simulink model "proj7_p1"  (R2016b)
settings: Solver=VariableStepAuto  StartTime=0.0  StopTime=10.0  RelTol=1e-3  EnableMultiTasking=on
undefined symbols (not defined in the file or in its folder): mc
settings Model: Creator=dave0651  LastModifiedBy=Jinesh
settings OptimizationCC: LifeSpan=inf
settings DebuggingCC: SFUnexpectedBacktrackingDiag=warning  SFNoUnconditionalDefaultTransitionDiag=warning  SFExecutionAtInitializationDiag=none
settings GRTTargetCC: TargetLangStandard=C89/C90 (ANSI)  GeneratePreprocessorConditionals=Disable all
settings ConfigComp: CovMetricSettings=dw  CovHtmlReporting=on  CovSaveCumulativeToWorkspaceVar=on  CovSaveSingleToWorkspaceVar=on  CovExternalEMLEnable=off

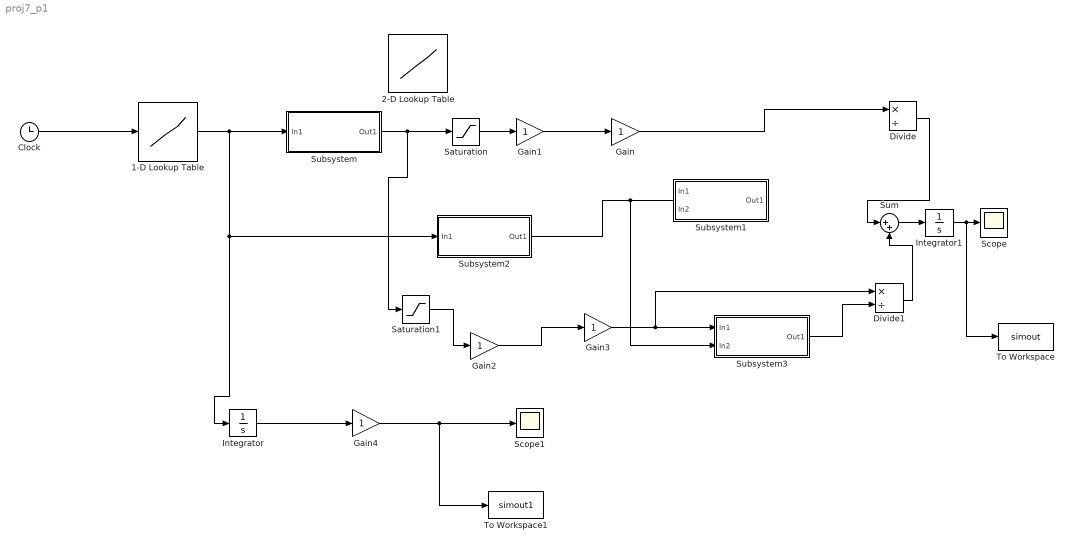
== system proj7_p1 ==
  1-D Lookup Table : Lookup_n-D  NumberOfTableDimensions=1  BreakpointsForDimension1=[-5:5]  Table=tanh([-5:5])  InternalRulePriority=Speed  RndMeth=Simplest  InputSameDT=on
  2-D Lookup Table : Lookup_n-D  BreakpointsForDimension1=[1:3]  BreakpointsForDimension2=[1:3]  InternalRulePriority=Speed  RndMeth=Simplest  InputSameDT=on
  Clock : Clock
  Divide : Product  Inputs=*/
  Divide1 : Product  Inputs=*/
  Gain{,1..4} (5 alike) : Gain
  Integrator : Integrator
  Integrator1 : Integrator
  Saturation : Saturate
  Saturation1 : Saturate
  Scope : Scope
  Scope1 : Scope
  Subsystem : Subsystem
  Subsystem1 : Subsystem
  Subsystem2 : Subsystem
  Subsystem3 : Subsystem
  Sum : Sum  Inputs=|++
  To Workspace : ToWorkspace  VariableName=simout  SaveFormat=Timeseries  SampleTime=-1
  To Workspace1 : ToWorkspace  VariableName=simout1  SaveFormat=Timeseries  SampleTime=-1
  wires:
  Integrator1/1 -> To Workspace/1, Scope/1
  Clock/1 -> 1-D Lookup Table/1
  1-D Lookup Table/1 -> Subsystem2/1(In1), Integrator/1, Subsystem/1(In1)
  Subsystem/1(Out1) -> Saturation1/1, Saturation/1
  Saturation/1 -> Gain1/1
  Gain1/1 -> Gain/1
  Gain/1 -> Divide/1
  Subsystem2/1(Out1) -> Subsystem3/2(In2)
  ? -> Divide/2
  Divide/1 -> Sum/1
  Sum/1 -> Integrator1/1
  Divide1/1 -> Sum/2
  Subsystem3/1(Out1) -> Divide1/2
  Gain2/1 -> Gain3/1
  Saturation1/1 -> Gain2/1
  Gain3/1 -> Divide1/1, Subsystem3/1(In1)
  Gain4/1 -> To Workspace1/1, Scope1/1
  Integrator/1 -> Gain4/1

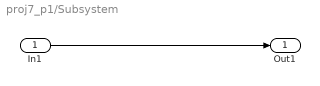
== system proj7_p1/Subsystem ==
  In1 : Inport
  Out1 : Outport
  wires:
  In1/1 -> Out1/1

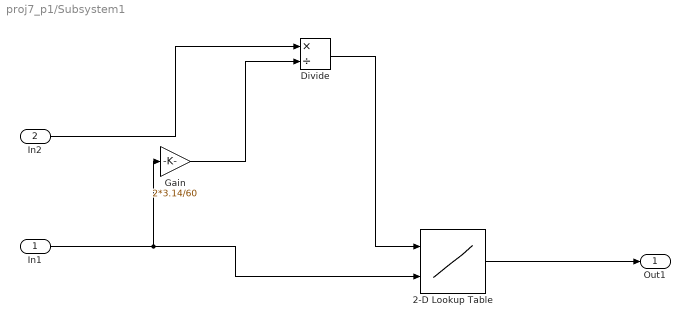
== system proj7_p1/Subsystem1 ==
  In1 : Inport
  In2 : Inport  Port=2
  2-D Lookup Table : Lookup_n-D  BreakpointsForDimension1=mc.trq_eff_index  BreakpointsForDimension2=mc.rpm_eff_index  Table=mc.eff_trq_map  InternalRulePriority=Speed  RndMeth=Simplest  InputSameDT=on
  Divide : Product  Inputs=*/
  Gain : Gain  Gain=2*3.14/60
  Out1 : Outport
  wires:
  In1/1 -> Gain/1, 2-D Lookup Table/2
  In2/1 -> Divide/1
  Gain/1 -> Divide/2
  Divide/1 -> 2-D Lookup Table/1
  2-D Lookup Table/1 -> Out1/1

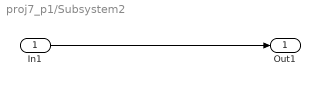
== system proj7_p1/Subsystem2 ==
  In1 : Inport
  Out1 : Outport
  wires:
  In1/1 -> Out1/1

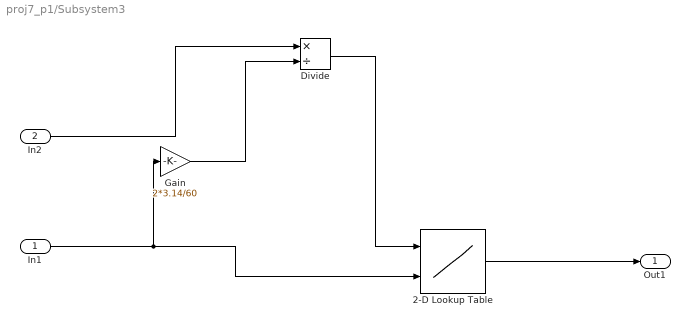
== system proj7_p1/Subsystem3 ==
  In1 : Inport
  In2 : Inport  Port=2
  2-D Lookup Table : Lookup_n-D  BreakpointsForDimension1=mc.trq_eff_index  BreakpointsForDimension2=mc.rpm_eff_index  Table=mc.eff_trq_map  InternalRulePriority=Speed  RndMeth=Simplest  InputSameDT=on
  Divide : Product  Inputs=*/
  Gain : Gain  Gain=2*3.14/60
  Out1 : Outport
  wires:
  In1/1 -> Gain/1, 2-D Lookup Table/2
  In2/1 -> Divide/1
  Gain/1 -> Divide/2
  Divide/1 -> 2-D Lookup Table/1
  2-D Lookup Table/1 -> Out1/1
